simulink model "pruebaImg"  (R2020a)
settings: Solver=FixedStepAuto  StartTime=0.0  StopTime=10.0  RelTol=1e-3
undefined symbols (not defined in the file): blue, blue2, blue3, green, green2, green3, red, red2, red3
libraries: simulink x3, androiduilib x1, androidaudiovideolib x1
settings Model: Creator=luisi  LastModifiedBy=luisi
settings OptimizationCC: EnhancedBackFolding=on  PassReuseOutputArgsAs=Individual arguments  ZeroExternalMemoryAtStartup=off  ZeroInternalMemoryAtStartup=off  MaxStackSize=64  OptimizeBlockOrder=speed  DifferentSizesBufferReuse=on  OptimizationCustomize=off  EfficientTunableParamExpr=on
settings DebuggingCC: ParameterTunabilityLossMsg=error
settings HardwareCC: ProdBitPerPointer=32  ProdBitPerSizeT=32  ProdBitPerPtrDiffT=32  ProdLargestAtomicInteger=Long  ProdLargestAtomicFloat=Double  ProdWordSize=32  ProdHWDeviceType=ARM Compatible->ARM Cortex
settings SFSimCC: MATLABDynamicMemAlloc=off
settings RTWCC: SystemTargetFile=ert.tlc  HardwareBoard=Android Device  TemplateMakefile=ert_default_tmf  RTWVerbose=off  Toolchain=Android SDK/NDK Tools
settings CodeAppCC: ForceParamTrailComments=on  IgnoreCustomStorageClasses=off  OperatorAnnotations=on  SimulinkDataObjDesc=on  SFDataObjDesc=on  InsertBlockDesc=on

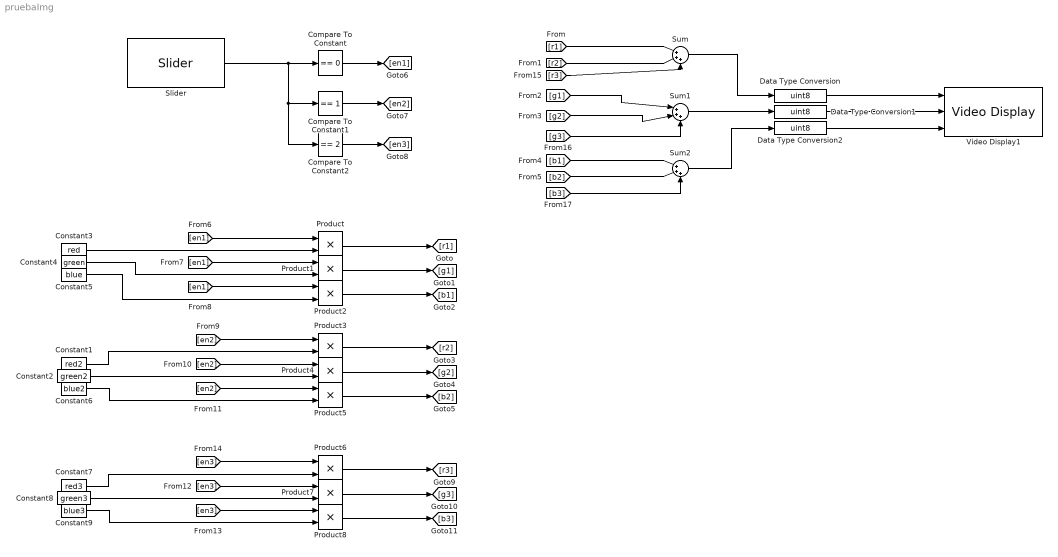
== system pruebaImg ==
  Compare To Constant : simulink/Logic and Bit Operations/Compare To Constant  relop===  const=0  OutDataTypeStr=uint8
  Compare To Constant1 : simulink/Logic and Bit Operations/Compare To Constant  relop===  const=1  OutDataTypeStr=uint8
  Compare To Constant2 : simulink/Logic and Bit Operations/Compare To Constant  relop===  const=2  OutDataTypeStr=uint8
  Constant1 : Constant  Value=red2
  Constant2 : Constant  Value=green2
  Constant3 : Constant  Value=red
  Constant4 : Constant  Value=green
  Constant5 : Constant  Value=blue
  Constant6 : Constant  Value=blue2
  Constant7 : Constant  Value=red3
  Constant8 : Constant  Value=green3
  Constant9 : Constant  Value=blue3
  Data Type Conversion : DataTypeConversion  OutDataTypeStr=uint8
  Data Type Conversion1 : DataTypeConversion  OutDataTypeStr=uint8
  Data Type Conversion2 : DataTypeConversion  OutDataTypeStr=uint8
  Product{,1..8} (9 alike) : Product
  Slider : androiduilib/Slider  Min=0  Value=0  Max=2  Resolution=1  SliderId=pruebaImg/Slider  SampleTime=0.1  BlockPlatform=Android
      settings: SourceProductBaseCode=ANDROID
  Sum : Sum  Inputs=|+++
  Sum1 : Sum  Inputs=|+++
  Sum2 : Sum  Inputs=|+++
  Video Display1 : androidaudiovideolib/Video Display  BlockPlatform=Android
      settings: SourceProductBaseCode=ANDROID
  wires:
  Data Type Conversion/1 -> Video Display1/1
  Data Type Conversion1/1 -> Video Display1/2
  Data Type Conversion2/1 -> Video Display1/3
  Constant3/1 -> Product/2
  Constant4/1 -> Product1/2
  Constant5/1 -> Product2/2
  Constant1/1 -> Product3/2
  Constant2/1 -> Product4/2
  Constant6/1 -> Product5/2
  Sum/1 -> Data Type Conversion/1
  Product/1 -> [r1]
  Product1/1 -> [g1]
  Product2/1 -> [b1]
  Product3/1 -> [r2]
  Product4/1 -> [g2]
  Product5/1 -> [b2]
  [r1] -> Sum/1
  [r2] -> Sum/2
  Sum1/1 -> Data Type Conversion1/1
  [g1] -> Sum1/1
  [g2] -> Sum1/2
  Sum2/1 -> Data Type Conversion2/1
  [b1] -> Sum2/1
  [b2] -> Sum2/2
  Compare To Constant/1 -> [en1]
  [en1] -> Product/1
  [en1] -> Product1/1
  [en1] -> Product2/1
  Compare To Constant1/1 -> [en2]
  [en2] -> Product3/1
  [en2] -> Product4/1
  [en2] -> Product5/1
  Compare To Constant2/1 -> [en3]
  Slider/1 -> Compare To Constant2/1, Compare To Constant1/1, Compare To Constant/1
  Product7/1 -> [g3]
  Product8/1 -> [b3]
  Constant7/1 -> Product6/2
  Constant8/1 -> Product7/2
  [en3] -> Product7/1
  Product6/1 -> [r3]
  Constant9/1 -> Product8/2
  [en3] -> Product6/1
  [en3] -> Product8/1
  [r3] -> Sum/3
  [g3] -> Sum1/3
  [b3] -> Sum2/3
